simulink model "corr_hw_test_tx"  (R2012b)
settings: Solver=ode45  StartTime=0.0  StopTime=200000  RelTol=1e-3
undefined symbols (not defined in the file or in its folder): gcbh, sfp, xlBlockLoadCallback
libraries: xbsIndex_r4 x2163, casper_library_misc x14, xps_library x6, ox_lib x1
(part 11 of 17)

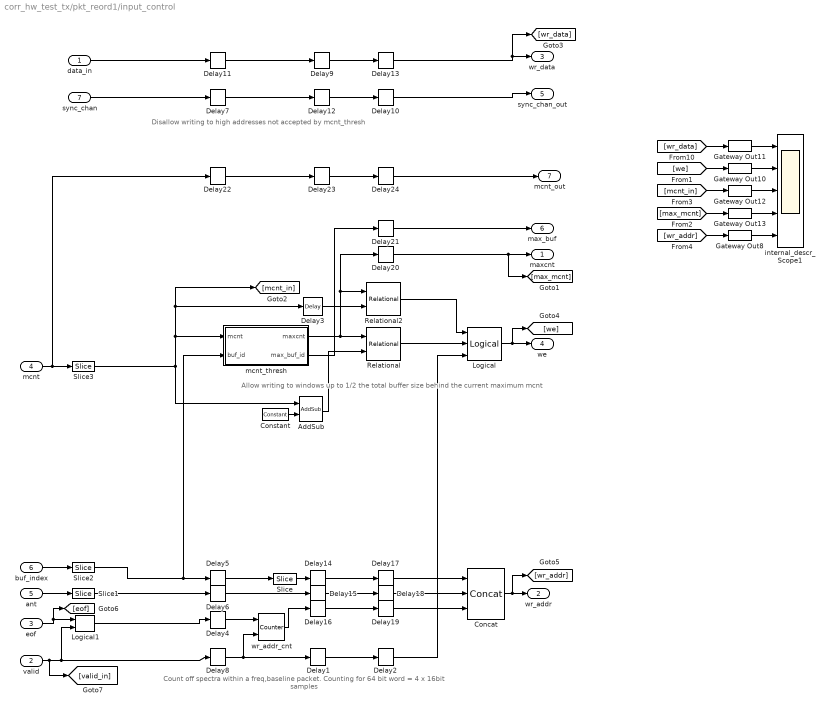
== system corr_hw_test_tx/pkt_reord1/input_control ==
  note: Allow writing to windows
      | up to 1/2 the total buffer size
      |  behind the current maximum mcnt
  note: Count off spectra
      | within a freq,baseline
      | packet.  Counting for
      | 64 bit word = 4 x 16bit samples
  note: Disallow writing to high addresses
      | not accepted by mcnt_thresh
  data_in : Inport
  valid : Inport  Port=2
  eof : Inport  Port=3
  mcnt : Inport  Port=4
  ant : Inport  Port=5
  buf_index : Inport  Port=6
  sync_chan : Inport  Port=7
  AddSub : xbsIndex_r4/AddSub  mode=Addition  use_carryin=off  use_carryout=off  en=off  latency=2  precision=User Defined  arith_type=Unsigned  n_bits=48 - ant_bits  bin_pt=0  quantization=Truncate  overflow=Wrap  dbl_ovrd=off  use_behavioral_HDL=on  hw_selection=Fabric  pipelined=off  use_rpm=on  block_type=addsub
      settings: xl_area=[0, 0, 0, 0, 0, 0, 0]  block_version=10.1.3
  Concat : xbsIndex_r4/Concat  num_inputs=3  dbl_ovrd=off  block_type=concat
      settings: block_version=10.1.3
  Constant : xbsIndex_r4/Constant  const=2^(window_bits - 1)  gui_display_data_type=Fixed-point  arith_type=Unsigned  n_bits=48 - xeng_bits  bin_pt=0  preci_type=Single  exp_width=8  frac_width=24  explicit_period=on  period=1  equ=P=C  opselect=C  inp2=PCIN>>17  opr=+  inp1=P  carry=CIN  dbl_ovrd=off  block_type=constant
  Delay{1,9,12,14..16,23} (7 alike) : xbsIndex_r4/Delay  rst=off  infoeditControl=Selection of Reset will increase slice count due to use of real FFs and instead of SRLs  en=off  latency=2  dbl_ovrd=off  reg_retiming=on  block_type=delay
      settings: xl_area=[0, 0, 0, 0, 0, 0, 0]
  Delay{2,4..8,10..11,13,17..22,24} (16 alike) : xbsIndex_r4/Delay  rst=off  infoeditControl=Selection of Reset will increase slice count due to use of real FFs and instead of SRLs  en=off  latency=1  dbl_ovrd=off  reg_retiming=on  block_type=delay
      settings: xl_area=[0, 0, 0, 0, 0, 0, 0]
  Delay3 : xbsIndex_r4/Delay  rst=off  infoeditControl=Selection of Reset will increase slice count due to use of real FFs and instead of SRLs  en=off  latency=2  dbl_ovrd=off  reg_retiming=off  block_type=delay
      settings: xl_area=[0, 0, 0, 0, 0, 0, 0]
  Gateway Out{8,10..13} (5 alike) : xbsIndex_r4/Gateway Out  inherit_from_input=off  hdl_port=off  timing_constraint=None  locs_specified=off  LOCs={}  UseAsDAC=off  DACChannel='1'  block_type=gatewayout
      settings: infoedit="Gateway out block.  Converts Xilinx fixed point inputs into ouputs of type Simulink integer, double, or fixed point.<P><P>Hardware notes:  In hardware these blocks become top level output ports or are discarded, depending on how they are configured."  xl_area=[0, 0, 0, 0, 0, 0, 0]  block_version=10.1.3
  Logical : xbsIndex_r4/Logical  logical_function=AND  inputs=3  en=off  latency=0  precision=Full  arith_type=Unsigned  n_bits=8  bin_pt=2  align_bp=on  dbl_ovrd=off  block_type=logical
      settings: xl_area=[0, 0, 0, 0, 0, 0, 0]
  Logical1 : xbsIndex_r4/Logical  logical_function=AND  inputs=2  en=off  latency=0  precision=Full  arith_type=Unsigned  n_bits=8  bin_pt=2  align_bp=on  dbl_ovrd=off  block_type=logical
      settings: xl_area=[0, 0, 0, 0, 0, 0, 0]
  Relational : xbsIndex_r4/Relational  mode=a<b  en=off  latency=1  dbl_ovrd=off  block_type=relational
      settings: xl_area=[0, 0, 0, 0, 0, 0, 0]  block_version=10.1.3
  Relational2 : xbsIndex_r4/Relational  mode=a>=b  en=off  latency=1  dbl_ovrd=off  block_type=relational
      settings: xl_area=[0, 0, 0, 0, 0, 0, 0]  block_version=10.1.3
  Slice : xbsIndex_r4/Slice  nbits=window_bits  boolean_output=off  mode=Lower Bit Location + Width  bit1=0  base1=MSB of Input  bit0=0  base0=LSB of Input  dbl_ovrd=off  block_type=slice
      settings: infoedit="Extracts a given range of bits from each input sample and presents it at the output.  The output type is ordinarily unsigned with binary point at zero, but can be Boolean when the slice is one bit wide.<P><P>Hardware notes: In hardware this block costs nothing."  block_version=10.1.3
  Slice1 : xbsIndex_r4/Slice  nbits=ant_bits  boolean_output=off  mode=Lower Bit Location + Width  bit1=0  base1=MSB of Input  bit0=0  base0=LSB of Input  dbl_ovrd=off  block_type=slice
      settings: infoedit="Extracts a given range of bits from each input sample and presents it at the output.  The output type is ordinarily unsigned with binary point at zero, but can be Boolean when the slice is one bit wide.<P><P>Hardware notes: In hardware this block costs nothing."  block_version=10.1.3
  Slice2 : xbsIndex_r4/Slice  nbits=window_bits  boolean_output=off  mode=Lower Bit Location + Width  bit1=0  base1=MSB of Input  bit0=0  base0=LSB of Input  dbl_ovrd=off  block_type=slice
      settings: block_version=10.1.3
  Slice3 : xbsIndex_r4/Slice  nbits=48-xeng_bits  boolean_output=off  mode=Lower Bit Location + Width  bit1=2  base1=LSB of Input  bit0=xeng_bits  base0=LSB of Input  dbl_ovrd=off  block_type=slice
      settings: block_version=10.1.3
  internal_descr_Scope1 : Scope  NumInputPorts=5
      settings: TimeRange=1  YMin=2.24317e+21~-1~7.6~7.6~7.6  YMax=2.47929e+21~1~8.4~8.4~8.4  SaveName=ScopeData5
  mcnt_thresh : Subsystem
  wr_addr_cnt : xbsIndex_r4/Counter  cnt_type=Free Running  cnt_to=Inf  operation=Up  start_count=0  cnt_by_val=1  arith_type=Unsigned  n_bits=x_int_bits + x_parallel_bits - 3  bin_pt=0  load_pin=off  rst=on  en=on  explicit_period=off  period=1  dbl_ovrd=off  use_behavioral_HDL=off  implementation=Fabric  use_rpm=on  block_type=counter
      settings: xl_area=[0, 0, 0, 0, 0, 0, 0]
  maxcnt : Outport
  wr_addr : Outport  Port=2
  wr_data : Outport  Port=3
  we : Outport  Port=4
  sync_chan_out : Outport  Port=5
  max_buf : Outport  Port=6
  mcnt_out : Outport  Port=7
  wires:
  Delay24/1 -> mcnt_out/1
  Delay23/1 -> Delay24/1
  Delay22/1 -> Delay23/1
  Delay21/1 -> max_buf/1
  mcnt_thresh/2(max_buf_id) -> Delay21/1
  sync_chan/1 -> Delay7/1
  Delay12/1 -> Delay10/1
  Delay10/1 -> sync_chan_out/1
  Delay7/1 -> Delay12/1
  Slice2/1 -> Delay5/1, mcnt_thresh/2(buf_id)
  buf_index/1 -> Slice2/1
  Slice3/1 -> AddSub/1, [mcnt_in], Delay3/1, mcnt_thresh/1(mcnt)
  Delay3/1 -> Relational2/2
  Relational2/1 -> Logical/1
  mcnt_thresh/1(maxcnt) -> Relational2/1, Delay20/1, Relational/1
  Constant/1 -> AddSub/2
  AddSub/1 -> Relational/2
  Slice/1 -> Delay14/1
  Slice1/1 -> Delay6/1
  wr_addr_cnt/1 -> Delay16/1
  valid/1 -> Delay8/1, Logical1/2, [valid_in]
  Relational/1 -> Logical/2
  Logical/1 -> we/1, [we]
  Delay2/1 -> Logical/3
  Delay4/1 -> wr_addr_cnt/1
  Delay8/1 -> wr_addr_cnt/2, Delay1/1
  mcnt/1 -> Slice3/1, Delay22/1
  ant/1 -> Slice1/1
  Logical1/1 -> Delay4/1
  eof/1 -> Logical1/1, [eof]
  Delay5/1 -> Slice/1
  Delay6/1 -> Delay15/1
  data_in/1 -> Delay11/1
  Delay9/1 -> Delay13/1
  Delay13/1 -> wr_data/1, [wr_data]
  Delay11/1 -> Delay9/1
  Concat/1 -> wr_addr/1, [wr_addr]
  Delay1/1 -> Delay2/1
  Delay16/1 -> Delay19/1
  Delay15/1 -> Delay18/1
  Delay14/1 -> Delay17/1
  Delay17/1 -> Concat/1
  Delay18/1 -> Concat/2
  Delay19/1 -> Concat/3
  Delay20/1 -> maxcnt/1, [max_mcnt]
  Gateway Out10/1 -> internal_descr_Scope1/2
  Gateway Out11/1 -> internal_descr_Scope1/1
  Gateway Out12/1 -> internal_descr_Scope1/3
  Gateway Out13/1 -> internal_descr_Scope1/4
  Gateway Out8/1 -> internal_descr_Scope1/5
  [wr_data] -> Gateway Out11/1
  [we] -> Gateway Out10/1
  [mcnt_in] -> Gateway Out12/1
  [max_mcnt] -> Gateway Out13/1
  [wr_addr] -> Gateway Out8/1

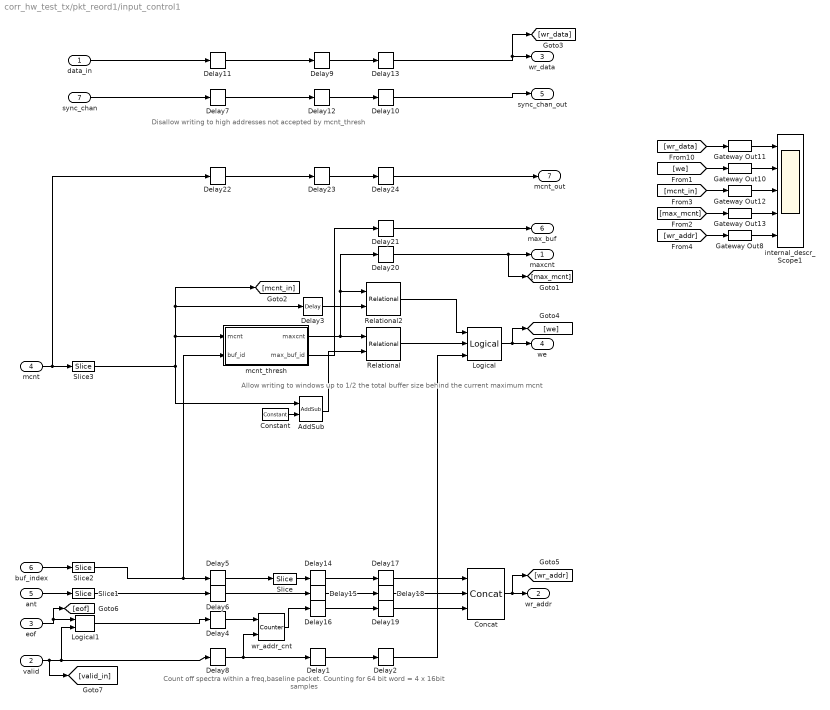
== system corr_hw_test_tx/pkt_reord1/input_control1 ==
  note: Disallow writing to high addresses
      | not accepted by mcnt_thresh
  note: Count off spectra
      | within a freq,baseline
      | packet.  Counting for
      | 64 bit word = 4 x 16bit samples
  note: Allow writing to windows
      | up to 1/2 the total buffer size
      |  behind the current maximum mcnt
  data_in : Inport
  valid : Inport  Port=2
  eof : Inport  Port=3
  mcnt : Inport  Port=4
  ant : Inport  Port=5
  buf_index : Inport  Port=6
  sync_chan : Inport  Port=7
  AddSub : xbsIndex_r4/AddSub  mode=Addition  use_carryin=off  use_carryout=off  en=off  latency=2  precision=User Defined  arith_type=Unsigned  n_bits=48 - ant_bits  bin_pt=0  quantization=Truncate  overflow=Wrap  dbl_ovrd=off  use_behavioral_HDL=on  hw_selection=Fabric  pipelined=off  use_rpm=on  block_type=addsub
      settings: xl_area=[0, 0, 0, 0, 0, 0, 0]  block_version=10.1.3
  Concat : xbsIndex_r4/Concat  num_inputs=3  dbl_ovrd=off  block_type=concat
      settings: block_version=10.1.3
  Constant : xbsIndex_r4/Constant  const=2^(window_bits - 1)  gui_display_data_type=Fixed-point  arith_type=Unsigned  n_bits=48 - xeng_bits  bin_pt=0  preci_type=Single  exp_width=8  frac_width=24  explicit_period=on  period=1  equ=P=C  opselect=C  inp2=PCIN>>17  opr=+  inp1=P  carry=CIN  dbl_ovrd=off  block_type=constant
  Delay{1,9,12,14..16,23} (7 alike) : xbsIndex_r4/Delay  rst=off  infoeditControl=Selection of Reset will increase slice count due to use of real FFs and instead of SRLs  en=off  latency=2  dbl_ovrd=off  reg_retiming=on  block_type=delay
      settings: xl_area=[0, 0, 0, 0, 0, 0, 0]
  Delay{2,4..8,10..11,13,17..22,24} (16 alike) : xbsIndex_r4/Delay  rst=off  infoeditControl=Selection of Reset will increase slice count due to use of real FFs and instead of SRLs  en=off  latency=1  dbl_ovrd=off  reg_retiming=on  block_type=delay
      settings: xl_area=[0, 0, 0, 0, 0, 0, 0]
  Delay3 : xbsIndex_r4/Delay  rst=off  infoeditControl=Selection of Reset will increase slice count due to use of real FFs and instead of SRLs  en=off  latency=2  dbl_ovrd=off  reg_retiming=off  block_type=delay
      settings: xl_area=[0, 0, 0, 0, 0, 0, 0]
  Gateway Out{8,10..13} (5 alike) : xbsIndex_r4/Gateway Out  inherit_from_input=off  hdl_port=off  timing_constraint=None  locs_specified=off  LOCs={}  UseAsDAC=off  DACChannel='1'  block_type=gatewayout
      settings: infoedit="Gateway out block.  Converts Xilinx fixed point inputs into ouputs of type Simulink integer, double, or fixed point.<P><P>Hardware notes:  In hardware these blocks become top level output ports or are discarded, depending on how they are configured."  xl_area=[0, 0, 0, 0, 0, 0, 0]  block_version=10.1.3
  Logical : xbsIndex_r4/Logical  logical_function=AND  inputs=3  en=off  latency=0  precision=Full  arith_type=Unsigned  n_bits=8  bin_pt=2  align_bp=on  dbl_ovrd=off  block_type=logical
      settings: xl_area=[0, 0, 0, 0, 0, 0, 0]
  Logical1 : xbsIndex_r4/Logical  logical_function=AND  inputs=2  en=off  latency=0  precision=Full  arith_type=Unsigned  n_bits=8  bin_pt=2  align_bp=on  dbl_ovrd=off  block_type=logical
      settings: xl_area=[0, 0, 0, 0, 0, 0, 0]
  Relational : xbsIndex_r4/Relational  mode=a<b  en=off  latency=1  dbl_ovrd=off  block_type=relational
      settings: xl_area=[0, 0, 0, 0, 0, 0, 0]  block_version=10.1.3
  Relational2 : xbsIndex_r4/Relational  mode=a>=b  en=off  latency=1  dbl_ovrd=off  block_type=relational
      settings: xl_area=[0, 0, 0, 0, 0, 0, 0]  block_version=10.1.3
  Slice : xbsIndex_r4/Slice  nbits=window_bits  boolean_output=off  mode=Lower Bit Location + Width  bit1=0  base1=MSB of Input  bit0=0  base0=LSB of Input  dbl_ovrd=off  block_type=slice
      settings: infoedit="Extracts a given range of bits from each input sample and presents it at the output.  The output type is ordinarily unsigned with binary point at zero, but can be Boolean when the slice is one bit wide.<P><P>Hardware notes: In hardware this block costs nothing."  block_version=10.1.3
  Slice1 : xbsIndex_r4/Slice  nbits=ant_bits  boolean_output=off  mode=Lower Bit Location + Width  bit1=0  base1=MSB of Input  bit0=0  base0=LSB of Input  dbl_ovrd=off  block_type=slice
      settings: infoedit="Extracts a given range of bits from each input sample and presents it at the output.  The output type is ordinarily unsigned with binary point at zero, but can be Boolean when the slice is one bit wide.<P><P>Hardware notes: In hardware this block costs nothing."  block_version=10.1.3
  Slice2 : xbsIndex_r4/Slice  nbits=window_bits  boolean_output=off  mode=Lower Bit Location + Width  bit1=0  base1=MSB of Input  bit0=0  base0=LSB of Input  dbl_ovrd=off  block_type=slice
      settings: block_version=10.1.3
  Slice3 : xbsIndex_r4/Slice  nbits=48-xeng_bits  boolean_output=off  mode=Lower Bit Location + Width  bit1=2  base1=LSB of Input  bit0=xeng_bits  base0=LSB of Input  dbl_ovrd=off  block_type=slice
      settings: block_version=10.1.3
  internal_descr_Scope1 : Scope  NumInputPorts=5
      settings: TimeRange=1  YMin=2.24317e+21~-1~7.6~7.6~7.6  YMax=2.47929e+21~1~8.4~8.4~8.4  SaveName=ScopeData5
  mcnt_thresh : Subsystem
  wr_addr_cnt : xbsIndex_r4/Counter  cnt_type=Free Running  cnt_to=Inf  operation=Up  start_count=0  cnt_by_val=1  arith_type=Unsigned  n_bits=x_int_bits + x_parallel_bits - 3  bin_pt=0  load_pin=off  rst=on  en=on  explicit_period=off  period=1  dbl_ovrd=off  use_behavioral_HDL=off  implementation=Fabric  use_rpm=on  block_type=counter
      settings: xl_area=[0, 0, 0, 0, 0, 0, 0]
  maxcnt : Outport
  wr_addr : Outport  Port=2
  wr_data : Outport  Port=3
  we : Outport  Port=4
  sync_chan_out : Outport  Port=5
  max_buf : Outport  Port=6
  mcnt_out : Outport  Port=7
  wires:
  [wr_addr] -> Gateway Out8/1
  [max_mcnt] -> Gateway Out13/1
  [mcnt_in] -> Gateway Out12/1
  [we] -> Gateway Out10/1
  [wr_data] -> Gateway Out11/1
  Gateway Out8/1 -> internal_descr_Scope1/5
  Gateway Out13/1 -> internal_descr_Scope1/4
  Gateway Out12/1 -> internal_descr_Scope1/3
  Gateway Out11/1 -> internal_descr_Scope1/1
  Gateway Out10/1 -> internal_descr_Scope1/2
  Delay20/1 -> [max_mcnt], maxcnt/1
  Delay19/1 -> Concat/3
  Delay18/1 -> Concat/2
  Delay17/1 -> Concat/1
  Delay14/1 -> Delay17/1
  Delay15/1 -> Delay18/1
  Delay16/1 -> Delay19/1
  Delay1/1 -> Delay2/1
  Concat/1 -> [wr_addr], wr_addr/1
  Delay11/1 -> Delay9/1
  Delay13/1 -> [wr_data], wr_data/1
  Delay9/1 -> Delay13/1
  data_in/1 -> Delay11/1
  Delay6/1 -> Delay15/1
  Delay5/1 -> Slice/1
  eof/1 -> [eof], Logical1/1
  Logical1/1 -> Delay4/1
  ant/1 -> Slice1/1
  mcnt/1 -> Delay22/1, Slice3/1
  Delay8/1 -> Delay1/1, wr_addr_cnt/2
  Delay4/1 -> wr_addr_cnt/1
  Delay2/1 -> Logical/3
  Logical/1 -> [we], we/1
  Relational/1 -> Logical/2
  valid/1 -> [valid_in], Logical1/2, Delay8/1
  wr_addr_cnt/1 -> Delay16/1
  Slice1/1 -> Delay6/1
  Slice/1 -> Delay14/1
  AddSub/1 -> Relational/2
  Constant/1 -> AddSub/2
  mcnt_thresh/1(maxcnt) -> Relational/1, Delay20/1, Relational2/1
  Relational2/1 -> Logical/1
  Delay3/1 -> Relational2/2
  Slice3/1 -> mcnt_thresh/1(mcnt), Delay3/1, [mcnt_in], AddSub/1
  buf_index/1 -> Slice2/1
  Slice2/1 -> mcnt_thresh/2(buf_id), Delay5/1
  Delay7/1 -> Delay12/1
  Delay10/1 -> sync_chan_out/1
  Delay12/1 -> Delay10/1
  sync_chan/1 -> Delay7/1
  mcnt_thresh/2(max_buf_id) -> Delay21/1
  Delay21/1 -> max_buf/1
  Delay22/1 -> Delay23/1
  Delay23/1 -> Delay24/1
  Delay24/1 -> mcnt_out/1

== system corr_hw_test_tx/pkt_reord1/mask_ant_rd_bits ==
  addr_in : Inport
  Concat : xbsIndex_r4/Concat  num_inputs=2  dbl_ovrd=off  block_type=concat
      settings: block_version=10.1.3
  Slice3 : xbsIndex_r4/Slice  nbits=x_int_bits + x_parallel_bits - 4  boolean_output=off  mode=Lower Bit Location + Width  bit1=0  base1=MSB of Input  bit0=0  base0=LSB of Input  dbl_ovrd=off  block_type=slice
      settings: block_version=10.1.3
  Slice4 : xbsIndex_r4/Slice  nbits=window_bits  boolean_output=off  mode=Upper Bit Location + Width  bit1=0  base1=MSB of Input  bit0=0  base0=LSB of Input  dbl_ovrd=off  block_type=slice
      settings: block_version=10.1.3
  addr_out : Outport
  wires:
  Slice3/1 -> Concat/2
  Slice4/1 -> Concat/1
  Concat/1 -> addr_out/1
  addr_in/1 -> Slice3/1, Slice4/1

== system corr_hw_test_tx/pkt_reord1/mask_ant_wr_bits ==
  addr_in : Inport
  Concat : xbsIndex_r4/Concat  num_inputs=2  dbl_ovrd=off  block_type=concat
      settings: block_version=10.1.3
  Slice3 : xbsIndex_r4/Slice  nbits=x_int_bits + x_parallel_bits - 3  boolean_output=off  mode=Lower Bit Location + Width  bit1=0  base1=MSB of Input  bit0=0  base0=LSB of Input  dbl_ovrd=off  block_type=slice
      settings: block_version=10.1.3
  Slice4 : xbsIndex_r4/Slice  nbits=window_bits  boolean_output=off  mode=Upper Bit Location + Width  bit1=0  base1=MSB of Input  bit0=0  base0=LSB of Input  dbl_ovrd=off  block_type=slice
      settings: block_version=10.1.3
  addr_out : Outport
  wires:
  addr_in/1 -> Slice4/1, Slice3/1
  Concat/1 -> addr_out/1
  Slice4/1 -> Concat/1
  Slice3/1 -> Concat/2

== system corr_hw_test_tx/pkt_reord1/pre_process ==
  data_in : Inport
  valid_in : Inport  Port=2
  eof_in : Inport  Port=3
  mcnt : Inport  Port=4
  ant_in : Inport  Port=5
  flag_in : Inport  Port=6
  buf_index_in : Inport  Port=7
  sync_this_chan : Inport  Port=8
  never : xbsIndex_r4/Constant  const=0  gui_display_data_type=Boolean  arith_type=Boolean  n_bits=16  bin_pt=14  preci_type=Single  exp_width=8  frac_width=24  explicit_period=on  period=1  equ=P=C  opselect=C  inp2=PCIN>>17  opr=+  inp1=P  carry=CIN  dbl_ovrd=off  block_type=constant
  data_out : Outport
  valid : Outport  Port=2
  eof_out : Outport  Port=3
  mcnt_out : Outport  Port=4
  ant_out : Outport  Port=5
  flag_out : Outport  Port=6
  buf_index : Outport  Port=7
  sync_this_chan_out : Outport  Port=8
  err : Outport  Port=9
  wires:
  sync_this_chan/1 -> sync_this_chan_out/1
  never/1 -> err/1
  buf_index_in/1 -> buf_index/1
  valid_in/1 -> valid/1
  eof_in/1 -> eof_out/1
  flag_in/1 -> flag_out/1
  ant_in/1 -> ant_out/1
  data_in/1 -> data_out/1
  mcnt/1 -> mcnt_out/1

== system corr_hw_test_tx/pkt_reord1/pre_process1 ==
  data_in : Inport
  valid_in : Inport  Port=2
  eof_in : Inport  Port=3
  mcnt : Inport  Port=4
  ant_in : Inport  Port=5
  flag_in : Inport  Port=6
  buf_index_in : Inport  Port=7
  sync_this_chan : Inport  Port=8
  never : xbsIndex_r4/Constant  const=0  gui_display_data_type=Boolean  arith_type=Boolean  n_bits=16  bin_pt=14  preci_type=Single  exp_width=8  frac_width=24  explicit_period=on  period=1  equ=P=C  opselect=C  inp2=PCIN>>17  opr=+  inp1=P  carry=CIN  dbl_ovrd=off  block_type=constant
  data_out : Outport
  valid : Outport  Port=2
  eof_out : Outport  Port=3
  mcnt_out : Outport  Port=4
  ant_out : Outport  Port=5
  flag_out : Outport  Port=6
  buf_index : Outport  Port=7
  sync_this_chan_out : Outport  Port=8
  err : Outport  Port=9
  wires:
  mcnt/1 -> mcnt_out/1
  data_in/1 -> data_out/1
  ant_in/1 -> ant_out/1
  flag_in/1 -> flag_out/1
  eof_in/1 -> eof_out/1
  valid_in/1 -> valid/1
  buf_index_in/1 -> buf_index/1
  never/1 -> err/1
  sync_this_chan/1 -> sync_this_chan_out/1

== system corr_hw_test_tx/pkt_reord2/ant_sel ==
  addr_in : Inport
  ant_id : Inport  Port=2
  re : Inport  Port=3
  Delay4 : xbsIndex_r4/Delay  rst=off  infoeditControl=Selection of Reset will increase slice count due to use of real FFs and instead of SRLs  en=off  latency=1  dbl_ovrd=off  reg_retiming=off  block_type=delay
      settings: xl_area=[0, 0, 0, 0, 0, 0, 0]
  Logical : xbsIndex_r4/Logical  logical_function=AND  inputs=2  en=off  latency=1  precision=Full  arith_type=Unsigned  n_bits=16  bin_pt=0  align_bp=on  dbl_ovrd=off  block_type=logical
  Relational : xbsIndex_r4/Relational  mode=a=b  en=off  latency=1  dbl_ovrd=off  block_type=relational
  Slice1 : xbsIndex_r4/Slice  nbits=ant_bits  boolean_output=off  mode=Lower Bit Location + Width  bit1=0  base1=MSB of Input  bit0=0  base0=LSB of Input  dbl_ovrd=off  block_type=slice
      settings: block_version=10.1.3
  Slice4 : xbsIndex_r4/Slice  nbits=ant_bits  boolean_output=off  mode=Lower Bit Location + Width  bit1=0  base1=MSB of Input  bit0=x_int_bits + x_parallel_bits - 4  base0=LSB of Input  dbl_ovrd=off  block_type=slice
      settings: block_version=10.1.3
  en_out : Outport
  wires:
  Slice4/1 -> Relational/1
  addr_in/1 -> Slice4/1
  ant_id/1 -> Slice1/1
  Slice1/1 -> Relational/2
  re/1 -> Delay4/1
  Relational/1 -> Logical/1
  Logical/1 -> en_out/1
  Delay4/1 -> Logical/2

== system corr_hw_test_tx/pkt_reord2/edge_detect ==
  in : Inport
  Delay : xbsIndex_r4/Delay  rst=off  infoeditControl=Selection of Reset will increase slice count due to use of real FFs and instead of SRLs  en=off  latency=1  dbl_ovrd=off  reg_retiming=off  block_type=delay
      settings: xl_area=[0, 0, 0, 0, 0, 0, 0]
  Inverter : xbsIndex_r4/Inverter  en=off  latency=0  dbl_ovrd=off  block_type=inv
      settings: xl_area=[0, 0, 0, 0, 0, 0, 0]
  edge_op : xbsIndex_r4/Logical  logical_function=NOR  inputs=2  en=off  latency=0  precision=Full  arith_type=Unsigned  n_bits=8  bin_pt=2  align_bp=on  dbl_ovrd=off  block_type=logical
      settings: xl_area=[0, 0, 0, 0, 0, 0, 0]
  out : Outport
  wires:
  Inverter/1 -> edge_op/1
  edge_op/1 -> out/1
  in/1 -> Inverter/1, Delay/1
  Delay/1 -> edge_op/2

== system corr_hw_test_tx/pkt_reord2/edge_detect1 ==
  in : Inport
  Delay : xbsIndex_r4/Delay  rst=off  infoeditControl=Selection of Reset will increase slice count due to use of real FFs and instead of SRLs  en=off  latency=1  dbl_ovrd=off  reg_retiming=off  block_type=delay
      settings: xl_area=[0, 0, 0, 0, 0, 0, 0]
  Inverter : xbsIndex_r4/Inverter  en=off  latency=0  dbl_ovrd=off  block_type=inv
      settings: xl_area=[0, 0, 0, 0, 0, 0, 0]
  edge_op : xbsIndex_r4/Logical  logical_function=NOR  inputs=2  en=off  latency=0  precision=Full  arith_type=Unsigned  n_bits=8  bin_pt=2  align_bp=on  dbl_ovrd=off  block_type=logical
      settings: xl_area=[0, 0, 0, 0, 0, 0, 0]
  out : Outport
  wires:
  Delay/1 -> edge_op/2
  in/1 -> Delay/1, Inverter/1
  edge_op/1 -> out/1
  Inverter/1 -> edge_op/1

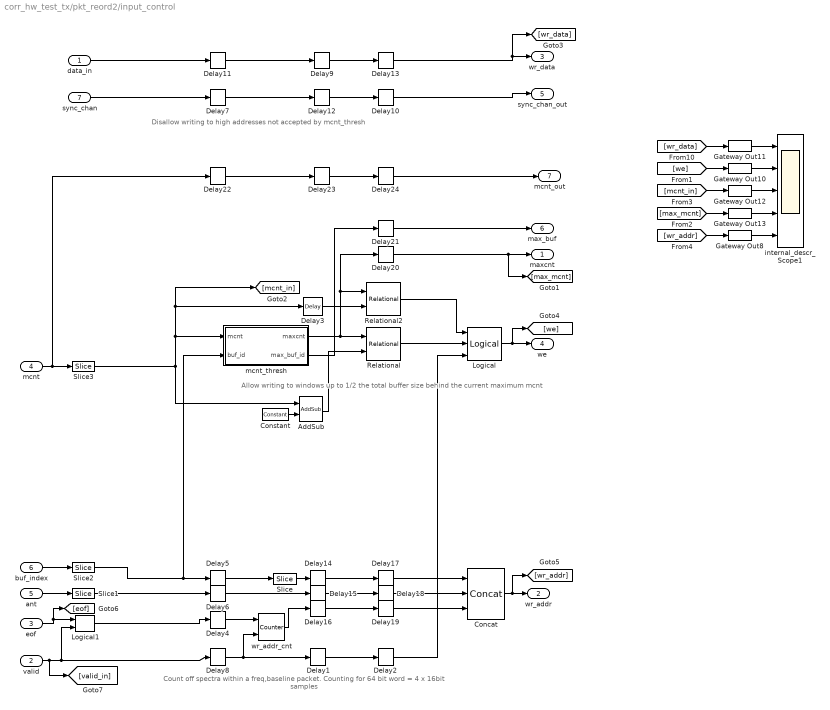
== system corr_hw_test_tx/pkt_reord2/input_control ==
  note: Disallow writing to high addresses
      | not accepted by mcnt_thresh
  note: Count off spectra
      | within a freq,baseline
      | packet.  Counting for
      | 64 bit word = 4 x 16bit samples
  note: Allow writing to windows
      | up to 1/2 the total buffer size
      |  behind the current maximum mcnt
  data_in : Inport
  valid : Inport  Port=2
  eof : Inport  Port=3
  mcnt : Inport  Port=4
  ant : Inport  Port=5
  buf_index : Inport  Port=6
  sync_chan : Inport  Port=7
  AddSub : xbsIndex_r4/AddSub  mode=Addition  use_carryin=off  use_carryout=off  en=off  latency=2  precision=User Defined  arith_type=Unsigned  n_bits=48 - ant_bits  bin_pt=0  quantization=Truncate  overflow=Wrap  dbl_ovrd=off  use_behavioral_HDL=on  hw_selection=Fabric  pipelined=off  use_rpm=on  block_type=addsub
      settings: xl_area=[0, 0, 0, 0, 0, 0, 0]  block_version=10.1.3
  Concat : xbsIndex_r4/Concat  num_inputs=3  dbl_ovrd=off  block_type=concat
      settings: block_version=10.1.3
  Constant : xbsIndex_r4/Constant  const=2^(window_bits - 1)  gui_display_data_type=Fixed-point  arith_type=Unsigned  n_bits=48 - xeng_bits  bin_pt=0  preci_type=Single  exp_width=8  frac_width=24  explicit_period=on  period=1  equ=P=C  opselect=C  inp2=PCIN>>17  opr=+  inp1=P  carry=CIN  dbl_ovrd=off  block_type=constant
  Delay{1,9,12,14..16,23} (7 alike) : xbsIndex_r4/Delay  rst=off  infoeditControl=Selection of Reset will increase slice count due to use of real FFs and instead of SRLs  en=off  latency=2  dbl_ovrd=off  reg_retiming=on  block_type=delay
      settings: xl_area=[0, 0, 0, 0, 0, 0, 0]
  Delay{2,4..8,10..11,13,17..22,24} (16 alike) : xbsIndex_r4/Delay  rst=off  infoeditControl=Selection of Reset will increase slice count due to use of real FFs and instead of SRLs  en=off  latency=1  dbl_ovrd=off  reg_retiming=on  block_type=delay
      settings: xl_area=[0, 0, 0, 0, 0, 0, 0]
  Delay3 : xbsIndex_r4/Delay  rst=off  infoeditControl=Selection of Reset will increase slice count due to use of real FFs and instead of SRLs  en=off  latency=2  dbl_ovrd=off  reg_retiming=off  block_type=delay
      settings: xl_area=[0, 0, 0, 0, 0, 0, 0]
  Gateway Out{8,10..13} (5 alike) : xbsIndex_r4/Gateway Out  inherit_from_input=off  hdl_port=off  timing_constraint=None  locs_specified=off  LOCs={}  UseAsDAC=off  DACChannel='1'  block_type=gatewayout
      settings: infoedit="Gateway out block.  Converts Xilinx fixed point inputs into ouputs of type Simulink integer, double, or fixed point.<P><P>Hardware notes:  In hardware these blocks become top level output ports or are discarded, depending on how they are configured."  xl_area=[0, 0, 0, 0, 0, 0, 0]  block_version=10.1.3
  Logical : xbsIndex_r4/Logical  logical_function=AND  inputs=3  en=off  latency=0  precision=Full  arith_type=Unsigned  n_bits=8  bin_pt=2  align_bp=on  dbl_ovrd=off  block_type=logical
      settings: xl_area=[0, 0, 0, 0, 0, 0, 0]
  Logical1 : xbsIndex_r4/Logical  logical_function=AND  inputs=2  en=off  latency=0  precision=Full  arith_type=Unsigned  n_bits=8  bin_pt=2  align_bp=on  dbl_ovrd=off  block_type=logical
      settings: xl_area=[0, 0, 0, 0, 0, 0, 0]
  Relational : xbsIndex_r4/Relational  mode=a<b  en=off  latency=1  dbl_ovrd=off  block_type=relational
      settings: xl_area=[0, 0, 0, 0, 0, 0, 0]  block_version=10.1.3
  Relational2 : xbsIndex_r4/Relational  mode=a>=b  en=off  latency=1  dbl_ovrd=off  block_type=relational
      settings: xl_area=[0, 0, 0, 0, 0, 0, 0]  block_version=10.1.3
  Slice : xbsIndex_r4/Slice  nbits=window_bits  boolean_output=off  mode=Lower Bit Location + Width  bit1=0  base1=MSB of Input  bit0=0  base0=LSB of Input  dbl_ovrd=off  block_type=slice
      settings: infoedit="Extracts a given range of bits from each input sample and presents it at the output.  The output type is ordinarily unsigned with binary point at zero, but can be Boolean when the slice is one bit wide.<P><P>Hardware notes: In hardware this block costs nothing."  block_version=10.1.3
  Slice1 : xbsIndex_r4/Slice  nbits=ant_bits  boolean_output=off  mode=Lower Bit Location + Width  bit1=0  base1=MSB of Input  bit0=0  base0=LSB of Input  dbl_ovrd=off  block_type=slice
      settings: infoedit="Extracts a given range of bits from each input sample and presents it at the output.  The output type is ordinarily unsigned with binary point at zero, but can be Boolean when the slice is one bit wide.<P><P>Hardware notes: In hardware this block costs nothing."  block_version=10.1.3
  Slice2 : xbsIndex_r4/Slice  nbits=window_bits  boolean_output=off  mode=Lower Bit Location + Width  bit1=0  base1=MSB of Input  bit0=0  base0=LSB of Input  dbl_ovrd=off  block_type=slice
      settings: block_version=10.1.3
  Slice3 : xbsIndex_r4/Slice  nbits=48-xeng_bits  boolean_output=off  mode=Lower Bit Location + Width  bit1=2  base1=LSB of Input  bit0=xeng_bits  base0=LSB of Input  dbl_ovrd=off  block_type=slice
      settings: block_version=10.1.3
  internal_descr_Scope1 : Scope  NumInputPorts=5
      settings: TimeRange=1  YMin=2.24317e+21~-1~7.6~7.6~7.6  YMax=2.47929e+21~1~8.4~8.4~8.4  SaveName=ScopeData5
  mcnt_thresh : Subsystem
  wr_addr_cnt : xbsIndex_r4/Counter  cnt_type=Free Running  cnt_to=Inf  operation=Up  start_count=0  cnt_by_val=1  arith_type=Unsigned  n_bits=x_int_bits + x_parallel_bits - 3  bin_pt=0  load_pin=off  rst=on  en=on  explicit_period=off  period=1  dbl_ovrd=off  use_behavioral_HDL=off  implementation=Fabric  use_rpm=on  block_type=counter
      settings: xl_area=[0, 0, 0, 0, 0, 0, 0]
  maxcnt : Outport
  wr_addr : Outport  Port=2
  wr_data : Outport  Port=3
  we : Outport  Port=4
  sync_chan_out : Outport  Port=5
  max_buf : Outport  Port=6
  mcnt_out : Outport  Port=7
  wires:
  [wr_addr] -> Gateway Out8/1
  [max_mcnt] -> Gateway Out13/1
  [mcnt_in] -> Gateway Out12/1
  [we] -> Gateway Out10/1
  [wr_data] -> Gateway Out11/1
  Gateway Out8/1 -> internal_descr_Scope1/5
  Gateway Out13/1 -> internal_descr_Scope1/4
  Gateway Out12/1 -> internal_descr_Scope1/3
  Gateway Out11/1 -> internal_descr_Scope1/1
  Gateway Out10/1 -> internal_descr_Scope1/2
  Delay20/1 -> [max_mcnt], maxcnt/1
  Delay19/1 -> Concat/3
  Delay18/1 -> Concat/2
  Delay17/1 -> Concat/1
  Delay14/1 -> Delay17/1
  Delay15/1 -> Delay18/1
  Delay16/1 -> Delay19/1
  Delay1/1 -> Delay2/1
  Concat/1 -> [wr_addr], wr_addr/1
  Delay11/1 -> Delay9/1
  Delay13/1 -> [wr_data], wr_data/1
  Delay9/1 -> Delay13/1
  data_in/1 -> Delay11/1
  Delay6/1 -> Delay15/1
  Delay5/1 -> Slice/1
  eof/1 -> [eof], Logical1/1
  Logical1/1 -> Delay4/1
  ant/1 -> Slice1/1
  mcnt/1 -> Delay22/1, Slice3/1
  Delay8/1 -> Delay1/1, wr_addr_cnt/2
  Delay4/1 -> wr_addr_cnt/1
  Delay2/1 -> Logical/3
  Logical/1 -> [we], we/1
  Relational/1 -> Logical/2
  valid/1 -> [valid_in], Logical1/2, Delay8/1
  wr_addr_cnt/1 -> Delay16/1
  Slice1/1 -> Delay6/1
  Slice/1 -> Delay14/1
  AddSub/1 -> Relational/2
  Constant/1 -> AddSub/2
  mcnt_thresh/1(maxcnt) -> Relational/1, Delay20/1, Relational2/1
  Relational2/1 -> Logical/1
  Delay3/1 -> Relational2/2
  Slice3/1 -> mcnt_thresh/1(mcnt), Delay3/1, [mcnt_in], AddSub/1
  buf_index/1 -> Slice2/1
  Slice2/1 -> mcnt_thresh/2(buf_id), Delay5/1
  Delay7/1 -> Delay12/1
  Delay10/1 -> sync_chan_out/1
  Delay12/1 -> Delay10/1
  sync_chan/1 -> Delay7/1
  mcnt_thresh/2(max_buf_id) -> Delay21/1
  Delay21/1 -> max_buf/1
  Delay22/1 -> Delay23/1
  Delay23/1 -> Delay24/1
  Delay24/1 -> mcnt_out/1

== system corr_hw_test_tx/pkt_reord2/input_control1 ==
  note: Allow writing to windows
      | up to 1/2 the total buffer size
      |  behind the current maximum mcnt
  note: Count off spectra
      | within a freq,baseline
      | packet.  Counting for
      | 64 bit word = 4 x 16bit samples
  note: Disallow writing to high addresses
      | not accepted by mcnt_thresh
  data_in : Inport
  valid : Inport  Port=2
  eof : Inport  Port=3
  mcnt : Inport  Port=4
  ant : Inport  Port=5
  buf_index : Inport  Port=6
  sync_chan : Inport  Port=7
  AddSub : xbsIndex_r4/AddSub  mode=Addition  use_carryin=off  use_carryout=off  en=off  latency=2  precision=User Defined  arith_type=Unsigned  n_bits=48 - ant_bits  bin_pt=0  quantization=Truncate  overflow=Wrap  dbl_ovrd=off  use_behavioral_HDL=on  hw_selection=Fabric  pipelined=off  use_rpm=on  block_type=addsub
      settings: xl_area=[0, 0, 0, 0, 0, 0, 0]  block_version=10.1.3
  Concat : xbsIndex_r4/Concat  num_inputs=3  dbl_ovrd=off  block_type=concat
      settings: block_version=10.1.3
  Constant : xbsIndex_r4/Constant  const=2^(window_bits - 1)  gui_display_data_type=Fixed-point  arith_type=Unsigned  n_bits=48 - xeng_bits  bin_pt=0  preci_type=Single  exp_width=8  frac_width=24  explicit_period=on  period=1  equ=P=C  opselect=C  inp2=PCIN>>17  opr=+  inp1=P  carry=CIN  dbl_ovrd=off  block_type=constant
  Delay{1,9,12,14..16,23} (7 alike) : xbsIndex_r4/Delay  rst=off  infoeditControl=Selection of Reset will increase slice count due to use of real FFs and instead of SRLs  en=off  latency=2  dbl_ovrd=off  reg_retiming=on  block_type=delay
      settings: xl_area=[0, 0, 0, 0, 0, 0, 0]
  Delay{2,4..8,10..11,13,17..22,24} (16 alike) : xbsIndex_r4/Delay  rst=off  infoeditControl=Selection of Reset will increase slice count due to use of real FFs and instead of SRLs  en=off  latency=1  dbl_ovrd=off  reg_retiming=on  block_type=delay
      settings: xl_area=[0, 0, 0, 0, 0, 0, 0]
  Delay3 : xbsIndex_r4/Delay  rst=off  infoeditControl=Selection of Reset will increase slice count due to use of real FFs and instead of SRLs  en=off  latency=2  dbl_ovrd=off  reg_retiming=off  block_type=delay
      settings: xl_area=[0, 0, 0, 0, 0, 0, 0]
  Gateway Out{8,10..13} (5 alike) : xbsIndex_r4/Gateway Out  inherit_from_input=off  hdl_port=off  timing_constraint=None  locs_specified=off  LOCs={}  UseAsDAC=off  DACChannel='1'  block_type=gatewayout
      settings: infoedit="Gateway out block.  Converts Xilinx fixed point inputs into ouputs of type Simulink integer, double, or fixed point.<P><P>Hardware notes:  In hardware these blocks become top level output ports or are discarded, depending on how they are configured."  xl_area=[0, 0, 0, 0, 0, 0, 0]  block_version=10.1.3
  Logical : xbsIndex_r4/Logical  logical_function=AND  inputs=3  en=off  latency=0  precision=Full  arith_type=Unsigned  n_bits=8  bin_pt=2  align_bp=on  dbl_ovrd=off  block_type=logical
      settings: xl_area=[0, 0, 0, 0, 0, 0, 0]
  Logical1 : xbsIndex_r4/Logical  logical_function=AND  inputs=2  en=off  latency=0  precision=Full  arith_type=Unsigned  n_bits=8  bin_pt=2  align_bp=on  dbl_ovrd=off  block_type=logical
      settings: xl_area=[0, 0, 0, 0, 0, 0, 0]
  Relational : xbsIndex_r4/Relational  mode=a<b  en=off  latency=1  dbl_ovrd=off  block_type=relational
      settings: xl_area=[0, 0, 0, 0, 0, 0, 0]  block_version=10.1.3
  Relational2 : xbsIndex_r4/Relational  mode=a>=b  en=off  latency=1  dbl_ovrd=off  block_type=relational
      settings: xl_area=[0, 0, 0, 0, 0, 0, 0]  block_version=10.1.3
  Slice : xbsIndex_r4/Slice  nbits=window_bits  boolean_output=off  mode=Lower Bit Location + Width  bit1=0  base1=MSB of Input  bit0=0  base0=LSB of Input  dbl_ovrd=off  block_type=slice
      settings: infoedit="Extracts a given range of bits from each input sample and presents it at the output.  The output type is ordinarily unsigned with binary point at zero, but can be Boolean when the slice is one bit wide.<P><P>Hardware notes: In hardware this block costs nothing."  block_version=10.1.3
  Slice1 : xbsIndex_r4/Slice  nbits=ant_bits  boolean_output=off  mode=Lower Bit Location + Width  bit1=0  base1=MSB of Input  bit0=0  base0=LSB of Input  dbl_ovrd=off  block_type=slice
      settings: infoedit="Extracts a given range of bits from each input sample and presents it at the output.  The output type is ordinarily unsigned with binary point at zero, but can be Boolean when the slice is one bit wide.<P><P>Hardware notes: In hardware this block costs nothing."  block_version=10.1.3
  Slice2 : xbsIndex_r4/Slice  nbits=window_bits  boolean_output=off  mode=Lower Bit Location + Width  bit1=0  base1=MSB of Input  bit0=0  base0=LSB of Input  dbl_ovrd=off  block_type=slice
      settings: block_version=10.1.3
  Slice3 : xbsIndex_r4/Slice  nbits=48-xeng_bits  boolean_output=off  mode=Lower Bit Location + Width  bit1=2  base1=LSB of Input  bit0=xeng_bits  base0=LSB of Input  dbl_ovrd=off  block_type=slice
      settings: block_version=10.1.3
  internal_descr_Scope1 : Scope  NumInputPorts=5
      settings: TimeRange=1  YMin=2.24317e+21~-1~7.6~7.6~7.6  YMax=2.47929e+21~1~8.4~8.4~8.4  SaveName=ScopeData5
  mcnt_thresh : Subsystem
  wr_addr_cnt : xbsIndex_r4/Counter  cnt_type=Free Running  cnt_to=Inf  operation=Up  start_count=0  cnt_by_val=1  arith_type=Unsigned  n_bits=x_int_bits + x_parallel_bits - 3  bin_pt=0  load_pin=off  rst=on  en=on  explicit_period=off  period=1  dbl_ovrd=off  use_behavioral_HDL=off  implementation=Fabric  use_rpm=on  block_type=counter
      settings: xl_area=[0, 0, 0, 0, 0, 0, 0]
  maxcnt : Outport
  wr_addr : Outport  Port=2
  wr_data : Outport  Port=3
  we : Outport  Port=4
  sync_chan_out : Outport  Port=5
  max_buf : Outport  Port=6
  mcnt_out : Outport  Port=7
  wires:
  Delay24/1 -> mcnt_out/1
  Delay23/1 -> Delay24/1
  Delay22/1 -> Delay23/1
  Delay21/1 -> max_buf/1
  mcnt_thresh/2(max_buf_id) -> Delay21/1
  sync_chan/1 -> Delay7/1
  Delay12/1 -> Delay10/1
  Delay10/1 -> sync_chan_out/1
  Delay7/1 -> Delay12/1
  Slice2/1 -> Delay5/1, mcnt_thresh/2(buf_id)
  buf_index/1 -> Slice2/1
  Slice3/1 -> AddSub/1, [mcnt_in], Delay3/1, mcnt_thresh/1(mcnt)
  Delay3/1 -> Relational2/2
  Relational2/1 -> Logical/1
  mcnt_thresh/1(maxcnt) -> Relational2/1, Delay20/1, Relational/1
  Constant/1 -> AddSub/2
  AddSub/1 -> Relational/2
  Slice/1 -> Delay14/1
  Slice1/1 -> Delay6/1
  wr_addr_cnt/1 -> Delay16/1
  valid/1 -> Delay8/1, Logical1/2, [valid_in]
  Relational/1 -> Logical/2
  Logical/1 -> we/1, [we]
  Delay2/1 -> Logical/3
  Delay4/1 -> wr_addr_cnt/1
  Delay8/1 -> wr_addr_cnt/2, Delay1/1
  mcnt/1 -> Slice3/1, Delay22/1
  ant/1 -> Slice1/1
  Logical1/1 -> Delay4/1
  eof/1 -> Logical1/1, [eof]
  Delay5/1 -> Slice/1
  Delay6/1 -> Delay15/1
  data_in/1 -> Delay11/1
  Delay9/1 -> Delay13/1
  Delay13/1 -> wr_data/1, [wr_data]
  Delay11/1 -> Delay9/1
  Concat/1 -> wr_addr/1, [wr_addr]
  Delay1/1 -> Delay2/1
  Delay16/1 -> Delay19/1
  Delay15/1 -> Delay18/1
  Delay14/1 -> Delay17/1
  Delay17/1 -> Concat/1
  Delay18/1 -> Concat/2
  Delay19/1 -> Concat/3
  Delay20/1 -> maxcnt/1, [max_mcnt]
  Gateway Out10/1 -> internal_descr_Scope1/2
  Gateway Out11/1 -> internal_descr_Scope1/1
  Gateway Out12/1 -> internal_descr_Scope1/3
  Gateway Out13/1 -> internal_descr_Scope1/4
  Gateway Out8/1 -> internal_descr_Scope1/5
  [wr_data] -> Gateway Out11/1
  [we] -> Gateway Out10/1
  [mcnt_in] -> Gateway Out12/1
  [max_mcnt] -> Gateway Out13/1
  [wr_addr] -> Gateway Out8/1

== system corr_hw_test_tx/pkt_reord2/mask_ant_rd_bits ==
  addr_in : Inport
  Concat : xbsIndex_r4/Concat  num_inputs=2  dbl_ovrd=off  block_type=concat
      settings: block_version=10.1.3
  Slice3 : xbsIndex_r4/Slice  nbits=x_int_bits + x_parallel_bits - 4  boolean_output=off  mode=Lower Bit Location + Width  bit1=0  base1=MSB of Input  bit0=0  base0=LSB of Input  dbl_ovrd=off  block_type=slice
      settings: block_version=10.1.3
  Slice4 : xbsIndex_r4/Slice  nbits=window_bits  boolean_output=off  mode=Upper Bit Location + Width  bit1=0  base1=MSB of Input  bit0=0  base0=LSB of Input  dbl_ovrd=off  block_type=slice
      settings: block_version=10.1.3
  addr_out : Outport
  wires:
  addr_in/1 -> Slice4/1, Slice3/1
  Concat/1 -> addr_out/1
  Slice4/1 -> Concat/1
  Slice3/1 -> Concat/2

== system corr_hw_test_tx/pkt_reord2/mask_ant_wr_bits ==
  addr_in : Inport
  Concat : xbsIndex_r4/Concat  num_inputs=2  dbl_ovrd=off  block_type=concat
      settings: block_version=10.1.3
  Slice3 : xbsIndex_r4/Slice  nbits=x_int_bits + x_parallel_bits - 3  boolean_output=off  mode=Lower Bit Location + Width  bit1=0  base1=MSB of Input  bit0=0  base0=LSB of Input  dbl_ovrd=off  block_type=slice
      settings: block_version=10.1.3
  Slice4 : xbsIndex_r4/Slice  nbits=window_bits  boolean_output=off  mode=Upper Bit Location + Width  bit1=0  base1=MSB of Input  bit0=0  base0=LSB of Input  dbl_ovrd=off  block_type=slice
      settings: block_version=10.1.3
  addr_out : Outport
  wires:
  Slice3/1 -> Concat/2
  Slice4/1 -> Concat/1
  Concat/1 -> addr_out/1
  addr_in/1 -> Slice3/1, Slice4/1

== system corr_hw_test_tx/pkt_reord2/pre_process ==
  data_in : Inport
  valid_in : Inport  Port=2
  eof_in : Inport  Port=3
  mcnt : Inport  Port=4
  ant_in : Inport  Port=5
  flag_in : Inport  Port=6
  buf_index_in : Inport  Port=7
  sync_this_chan : Inport  Port=8
  never : xbsIndex_r4/Constant  const=0  gui_display_data_type=Boolean  arith_type=Boolean  n_bits=16  bin_pt=14  preci_type=Single  exp_width=8  frac_width=24  explicit_period=on  period=1  equ=P=C  opselect=C  inp2=PCIN>>17  opr=+  inp1=P  carry=CIN  dbl_ovrd=off  block_type=constant
  data_out : Outport
  valid : Outport  Port=2
  eof_out : Outport  Port=3
  mcnt_out : Outport  Port=4
  ant_out : Outport  Port=5
  flag_out : Outport  Port=6
  buf_index : Outport  Port=7
  sync_this_chan_out : Outport  Port=8
  err : Outport  Port=9
  wires:
  mcnt/1 -> mcnt_out/1
  data_in/1 -> data_out/1
  ant_in/1 -> ant_out/1
  flag_in/1 -> flag_out/1
  eof_in/1 -> eof_out/1
  valid_in/1 -> valid/1
  buf_index_in/1 -> buf_index/1
  never/1 -> err/1
  sync_this_chan/1 -> sync_this_chan_out/1

== system corr_hw_test_tx/pkt_reord2/pre_process1 ==
  data_in : Inport
  valid_in : Inport  Port=2
  eof_in : Inport  Port=3
  mcnt : Inport  Port=4
  ant_in : Inport  Port=5
  flag_in : Inport  Port=6
  buf_index_in : Inport  Port=7
  sync_this_chan : Inport  Port=8
  never : xbsIndex_r4/Constant  const=0  gui_display_data_type=Boolean  arith_type=Boolean  n_bits=16  bin_pt=14  preci_type=Single  exp_width=8  frac_width=24  explicit_period=on  period=1  equ=P=C  opselect=C  inp2=PCIN>>17  opr=+  inp1=P  carry=CIN  dbl_ovrd=off  block_type=constant
  data_out : Outport
  valid : Outport  Port=2
  eof_out : Outport  Port=3
  mcnt_out : Outport  Port=4
  ant_out : Outport  Port=5
  flag_out : Outport  Port=6
  buf_index : Outport  Port=7
  sync_this_chan_out : Outport  Port=8
  err : Outport  Port=9
  wires:
  sync_this_chan/1 -> sync_this_chan_out/1
  never/1 -> err/1
  buf_index_in/1 -> buf_index/1
  valid_in/1 -> valid/1
  eof_in/1 -> eof_out/1
  flag_in/1 -> flag_out/1
  ant_in/1 -> ant_out/1
  data_in/1 -> data_out/1
  mcnt/1 -> mcnt_out/1

== system corr_hw_test_tx/pkt_reord3/ant_sel ==
  addr_in : Inport
  ant_id : Inport  Port=2
  re : Inport  Port=3
  Delay4 : xbsIndex_r4/Delay  rst=off  infoeditControl=Selection of Reset will increase slice count due to use of real FFs and instead of SRLs  en=off  latency=1  dbl_ovrd=off  reg_retiming=off  block_type=delay
      settings: xl_area=[0, 0, 0, 0, 0, 0, 0]
  Logical : xbsIndex_r4/Logical  logical_function=AND  inputs=2  en=off  latency=1  precision=Full  arith_type=Unsigned  n_bits=16  bin_pt=0  align_bp=on  dbl_ovrd=off  block_type=logical
  Relational : xbsIndex_r4/Relational  mode=a=b  en=off  latency=1  dbl_ovrd=off  block_type=relational
  Slice1 : xbsIndex_r4/Slice  nbits=ant_bits  boolean_output=off  mode=Lower Bit Location + Width  bit1=0  base1=MSB of Input  bit0=0  base0=LSB of Input  dbl_ovrd=off  block_type=slice
      settings: block_version=10.1.3
  Slice4 : xbsIndex_r4/Slice  nbits=ant_bits  boolean_output=off  mode=Lower Bit Location + Width  bit1=0  base1=MSB of Input  bit0=x_int_bits + x_parallel_bits - 4  base0=LSB of Input  dbl_ovrd=off  block_type=slice
      settings: block_version=10.1.3
  en_out : Outport
  wires:
  Delay4/1 -> Logical/2
  Logical/1 -> en_out/1
  Relational/1 -> Logical/1
  re/1 -> Delay4/1
  Slice1/1 -> Relational/2
  ant_id/1 -> Slice1/1
  addr_in/1 -> Slice4/1
  Slice4/1 -> Relational/1

== system corr_hw_test_tx/pkt_reord3/edge_detect ==
  in : Inport
  Delay : xbsIndex_r4/Delay  rst=off  infoeditControl=Selection of Reset will increase slice count due to use of real FFs and instead of SRLs  en=off  latency=1  dbl_ovrd=off  reg_retiming=off  block_type=delay
      settings: xl_area=[0, 0, 0, 0, 0, 0, 0]
  Inverter : xbsIndex_r4/Inverter  en=off  latency=0  dbl_ovrd=off  block_type=inv
      settings: xl_area=[0, 0, 0, 0, 0, 0, 0]
  edge_op : xbsIndex_r4/Logical  logical_function=NOR  inputs=2  en=off  latency=0  precision=Full  arith_type=Unsigned  n_bits=8  bin_pt=2  align_bp=on  dbl_ovrd=off  block_type=logical
      settings: xl_area=[0, 0, 0, 0, 0, 0, 0]
  out : Outport
  wires:
  Delay/1 -> edge_op/2
  in/1 -> Delay/1, Inverter/1
  edge_op/1 -> out/1
  Inverter/1 -> edge_op/1

== system corr_hw_test_tx/pkt_reord3/edge_detect1 ==
  in : Inport
  Delay : xbsIndex_r4/Delay  rst=off  infoeditControl=Selection of Reset will increase slice count due to use of real FFs and instead of SRLs  en=off  latency=1  dbl_ovrd=off  reg_retiming=off  block_type=delay
      settings: xl_area=[0, 0, 0, 0, 0, 0, 0]
  Inverter : xbsIndex_r4/Inverter  en=off  latency=0  dbl_ovrd=off  block_type=inv
      settings: xl_area=[0, 0, 0, 0, 0, 0, 0]
  edge_op : xbsIndex_r4/Logical  logical_function=NOR  inputs=2  en=off  latency=0  precision=Full  arith_type=Unsigned  n_bits=8  bin_pt=2  align_bp=on  dbl_ovrd=off  block_type=logical
      settings: xl_area=[0, 0, 0, 0, 0, 0, 0]
  out : Outport
  wires:
  Inverter/1 -> edge_op/1
  edge_op/1 -> out/1
  in/1 -> Inverter/1, Delay/1
  Delay/1 -> edge_op/2
